simulink library "Yaw_Ideal_Actuator_Lib"  (R2019b)
settings: Solver=ode45  StartTime=0.0  StopTime=10.0  RelTol=1e-3  EnableMultiTasking=on
undefined symbols (not defined in the file): deg, s, WT_Params
libraries: mblibv1 x1
Description:
  | Copyright 2009-2017 The MathWorks, Inc. MathWorks, Inc.
settings Model: Creator=smiller  LastModifiedBy=bhisma
settings DataIOCC: LimitDataPoints=on  SaveFormat=Array  SignalLoggingSaveFormat=ModelDataLogs  ReturnWorkspaceOutputs=off
settings OptimizationCC: ExpressionDepthLimit=2147483647  LifeSpan=inf
settings DebuggingCC: UnderspecifiedInitializationDetection=Classic  MergeDetectMultiDrivingBlocksExec=none  SolverPrmCheckMsg=warning  FcnCallInpInsideContextMsg=warning  AllowSymbolicDim=off  StateNameClashWarn=warning  SFUnexpectedBacktrackingDiag=warning  SFNoUnconditionalDefaultTransitionDiag=warning  SFExecutionAtInitializationDiag=none  ArithmeticOperatorsInVariantConditions=warning
settings HardwareCC: ProdBitPerPointer=32  ProdBitPerSizeT=32  ProdBitPerPtrDiffT=32  ProdLargestAtomicFloat=None  ProdIntDivRoundTo=Undefined  ProdEndianess=Unspecified  ProdWordSize=32  ProdHWDeviceType=32-bit Generic
settings ModelReferenceCC: PropagateSignalLabelsOutOfModel=off
settings SFSimCC: SimUseLocalCustomCode=off  CustomCodeUndefinedFunction=UseInterfaceOnly
settings RTWCC: RTWUseLocalCustomCode=off
settings CodeAppCC: StateflowObjectComments=on
settings GRTTargetCC: TargetLangStandard=C89/C90 (ANSI)  GeneratePreprocessorConditionals=Disable all  CombineOutputUpdateFcns=off  GRTInterface=on
settings ConfigComp: CovMetricSettings=dw  CovHtmlReporting=on  CovSaveCumulativeToWorkspaceVar=on  CovSaveSingleToWorkspaceVar=on  CovExternalEMLEnable=off  CovSFcnEnable=off

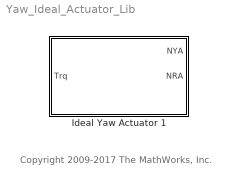
== system Yaw_Ideal_Actuator_Lib ==
  note: Copyright 2009-2017 The MathWorks, Inc.
  Ideal Yaw Actuator 1 : Subsystem
      mask Display: image(imread('Yaw_Ideal_Actuator_Horizontal_IMAGE.jpg'));

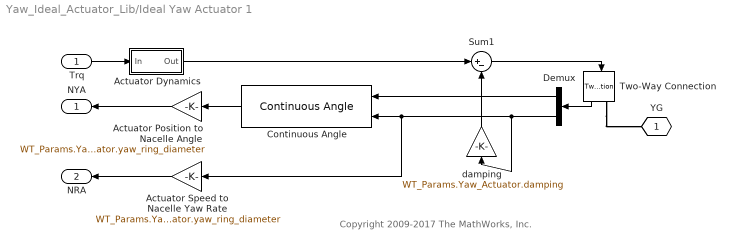
== system Yaw_Ideal_Actuator_Lib/Ideal Yaw Actuator 1 ==
  note: Copyright 2009-2017 The MathWorks, Inc.
  Trq : Inport
  Actuator Dynamics : Subsystem  mask(First-order lag supporting vector signals){b=WT_Params.Yaw_Actuator.ideal_actuator_time_constant, x_initial=0}
      mask prompts: b "Filter time constant"; x_initial "Initial output"
      mask help: Models a lag of the form 1/(b*s+1) where s is the Laplace operator.
  Actuator Position to Nacelle Angle : Gain  Gain=WT_Params.Yaw_Actuator.yaw_gear_diameter/WT_Params.Yaw_Actuator.yaw_ring_diameter
  Actuator Speed to Nacelle Yaw Rate : Gain  Gain=WT_Params.Yaw_Actuator.yaw_gear_diameter/WT_Params.Yaw_Actuator.yaw_ring_diameter
  Continuous Angle : mblibv1/Utilities/Continuous Angle  rad=deg  rads=deg/s
      settings: SourceProductName=Simscape Multibody  SourceProductBaseCode=MS
  Demux : Demux  Outputs=2
  Sum1 : Sum  Inputs=|+-
  Two-Way Connection : TwoWayConnection
  damping : Gain  Gain=WT_Params.Yaw_Actuator.damping
  YG : PMIOPort  Tag=PMCPort  Side=Right
  NYA : Outport
  NRA : Outport  Port=2
  wires:
  damping/1 -> Sum1/2
  Demux/2 -> damping/1, Continuous Angle/2, Actuator Speed to Nacelle Yaw Rate/1
  Demux/1 -> Continuous Angle/1
  Continuous Angle/1 -> Actuator Position to Nacelle Angle/1
  Actuator Position to Nacelle Angle/1 -> NYA/1
  Actuator Speed to Nacelle Yaw Rate/1 -> NRA/1
  Trq/1 -> Actuator Dynamics/1(In)
  Actuator Dynamics/1(Out) -> Sum1/1
  Sum1/1 -> Two-Way Connection/1
  Two-Way Connection/1 -> Demux/1
  connections:
  Two-Way Connection/RConn1 -- YG/RConn1

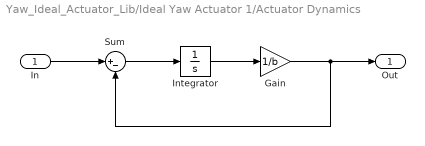
== system Yaw_Ideal_Actuator_Lib/Ideal Yaw Actuator 1/Actuator Dynamics ==
  In : Inport
  Gain : Gain  Gain=1/b
  Integrator : Integrator  InitialCondition=x_initial
  Sum : Sum  Inputs=|+-  SaturateOnIntegerOverflow=on  InputSameDT=on  OutDataTypeStr=Inherit: Same as first input
  Out : Outport
  wires:
  Sum/1 -> Integrator/1
  In/1 -> Sum/1
  Integrator/1 -> Gain/1
  Gain/1 -> Sum/2, Out/1
